simulink model "FourAgentsSinusoidal"  (R2021b)
settings: Solver=VariableStepAuto  StartTime=0.0  StopTime=50.0  RelTol=1e-3
settings Model: Creator=sharmin  LastModifiedBy=sharmin

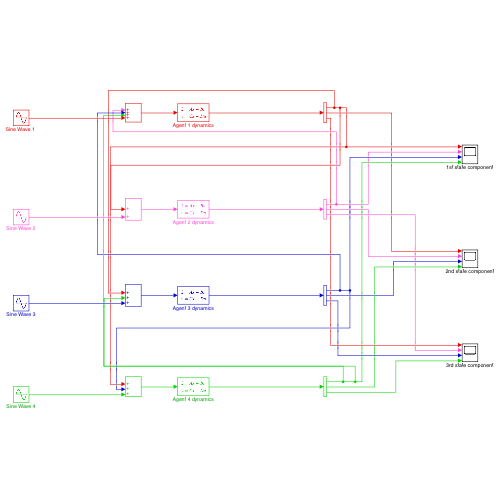
[thumbnail: Simulink's stored preview of the top-level diagram]
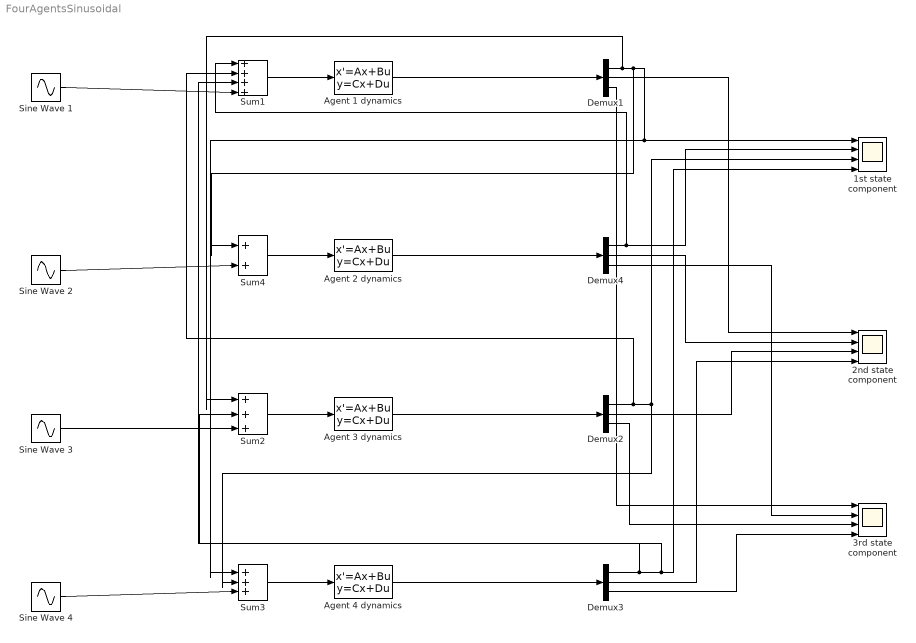
== system FourAgentsSinusoidal ==
  1st state component : Scope  NumInputPorts=4
  2nd state component : Scope  NumInputPorts=4
  3rd state component : Scope  NumInputPorts=4
  Agent 1 dynamics : StateSpace  A=[0 1 0; 0 0 1; -3 -4 -6]  B=[0; 0 ; 1]  C=eye(3)  D=zeros(3,1)  InitialCondition=[1 1 1]  AllowTunableDMatrix=on
  Agent 2 dynamics : StateSpace  A=[0 1 0; 0 0 1; -1 -4 -6]  B=[0; 0 ; 1]  C=eye(3)  D=zeros(3,1)  InitialCondition=[2 2 2]  AllowTunableDMatrix=on
  Agent 3 dynamics : StateSpace  A=[0 1 0; 0 0 1; -2 -4 -6]  B=[0; 0 ; 1]  C=eye(3)  D=zeros(3,1)  InitialCondition=[3 3 3]  AllowTunableDMatrix=on
  Agent 4 dynamics : StateSpace  A=[0 1 0; 0 0 1; -2 -4 -6]  B=[0; 0 ; 1]  C=eye(3)  D=zeros(3,1)  InitialCondition=[4 4 4]  AllowTunableDMatrix=on
  Demux{1..4} (4 alike) : Demux  Outputs=3
  "Sine Wave 1 " : Sin  SampleTime=0
  Sine Wave 2 : Sin  SampleTime=0
  Sine Wave 3 : Sin  SampleTime=0
  Sine Wave 4 : Sin  SampleTime=0
  Sum1 : Sum  Inputs=|++++
  Sum2 : Sum  Inputs=|+++
  Sum3 : Sum  Inputs=|+++
  Sum4 : Sum  Inputs=|++
  wires:
  Agent 1 dynamics/1 -> Demux1/1
  Sum1/1 -> Agent 1 dynamics/1
  Agent 2 dynamics/1 -> Demux4/1
  Sum4/1 -> Agent 2 dynamics/1
  Sum2/1 -> Agent 3 dynamics/1
  Agent 3 dynamics/1 -> Demux2/1
  Sum3/1 -> Agent 4 dynamics/1
  Agent 4 dynamics/1 -> Demux3/1
  Demux1/1 -> Sum2/1, Sum4/1, Sum3/1, 1st state component/1
  Demux4/1 -> Sum1/1, 1st state component/2
  Demux2/1 -> Sum1/2, 1st state component/3, Sum3/2
  Demux3/1 -> 1st state component/4, Sum2/2, Sum1/3
  Demux1/2 -> 2nd state component/1
  Demux4/2 -> 2nd state component/2
  Demux2/2 -> 2nd state component/3
  Demux3/2 -> 2nd state component/4
  Demux1/3 -> 3rd state component/1
  Demux4/3 -> 3rd state component/2
  Demux2/3 -> 3rd state component/3
  Demux3/3 -> 3rd state component/4
  Sine Wave 2/1 -> Sum4/2
  "Sine Wave 1 "/1 -> Sum1/4
  Sine Wave 3/1 -> Sum2/3
  Sine Wave 4/1 -> Sum3/3
